simulink model "exp4_1"  (R2024b)
settings: Solver=VariableStepAuto  StartTime=0.0  StopTime=10  RelTol=1e-3
InitFcn:
  | Voc=32.9;
  | Iscn=8.21;
  | k=1.38e-23;
  | Ns=54;
  | Np=1;
  | G=524;
  | Gn=1000;
  | Kv=-0.1230;
  | Ki=0.0032;
  | T=301;
  | Tn=300;
  | q=1.6e-19;
  | I0n=9.85e-8;
  | Eg=1.12;
  | Ign=8.214;
  | Rs=0.221;
  | Rp=414.5;
  | a=1.0;
libraries: spsSeriesRLCBranchLib x6, spsVoltageMeasurementLib x4, spsCurrentMeasurementLib x3, spsDiodeLib x2, spsFirstOrderFilterLib x2, spsMeanLib x2, slpidlib x1, spsMosfetLib x1, spsControlledCurrentSourceLib x1, simulink x1, spspowerguiLib x1, spsPWMGeneratorDCDCLib x1
settings Model: Creator=palla  LastModifiedBy=palla

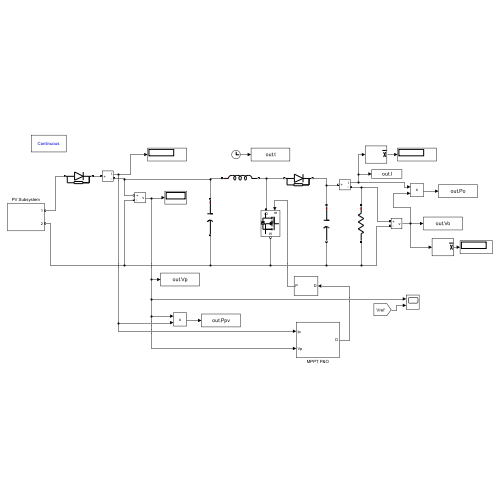
[thumbnail: Simulink's stored preview of the top-level diagram]
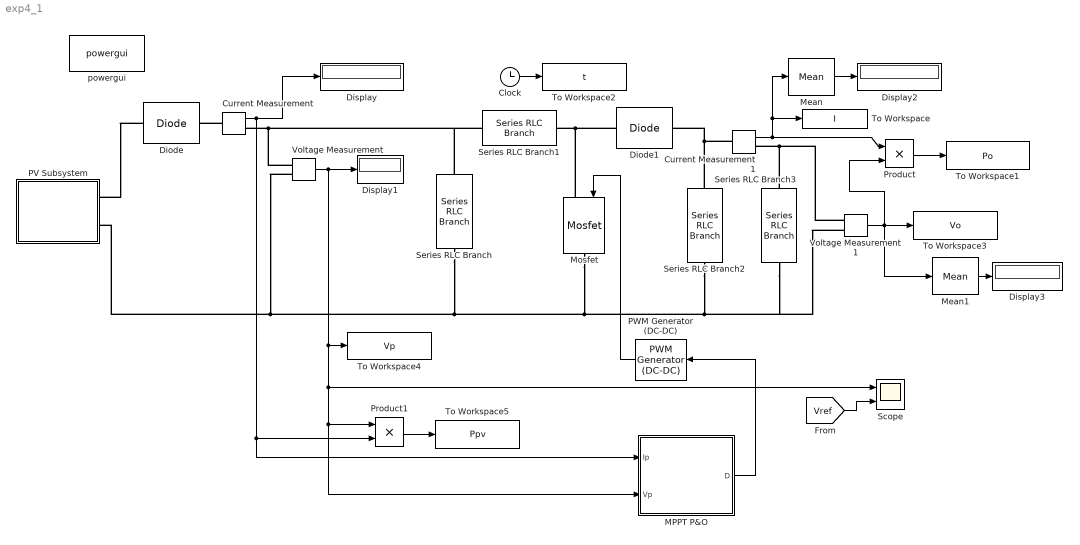
== system exp4_1 ==
  Clock : Clock
  Current Measurement : spsCurrentMeasurementLib/Current Measurement  PhasorSimulation=off  OutputType=Complex  PSBequivalent=0
  Current Measurement1 : spsCurrentMeasurementLib/Current Measurement  PhasorSimulation=off  OutputType=Complex  PSBequivalent=0
  Diode : spsDiodeLib/Diode  Ron=0.001  Lon=0  Vf=0.8  IC=0  UseSnubber=0  Rs=500  Cs=250e-9  Measurements=off
  Diode1 : spsDiodeLib/Diode  Ron=0.001  Lon=0  Vf=0.8  IC=0  UseSnubber=0  Rs=500  Cs=250e-9  Measurements=off
  Display{,1..3} (4 alike) : Display
  MPPT P&O : Subsystem
  Mean : spsMeanLib/Mean  Freq=60  Vinit=0  Ts=0
  Mean1 : spsMeanLib/Mean  Freq=60  Vinit=0  Ts=0
  Mosfet : spsMosfetLib/Mosfet  Ron=0.1  Lon=0  Rd=0.01  Vfd=0  IC=0  Rs=1e5  Cs=inf  Measurements=off
  PV Subsystem : Subsystem
  PWM Generator (DC-DC) : spsPWMGeneratorDCDCLib/PWM Generator (DC-DC)  Fsw=5000  Ts=0
  Product : Product
  Product1 : Product
  Scope : Scope  NumInputPorts=2
  Series RLC Branch : spsSeriesRLCBranchLib/Series RLC Branch  LConnTagsString=__new0  RConnTagsString=__new0  BranchType=C  Resistance=1  Inductance=1e-3  SetiL0=off  InitialCurrent=0  Capacitance=110e-6  Setx0=off  InitialVoltage=0  Measurements=None
  Series RLC Branch1 : spsSeriesRLCBranchLib/Series RLC Branch  LConnTagsString=__new0  RConnTagsString=__new0  BranchType=L  Resistance=1  Inductance=0.01025  SetiL0=off  InitialCurrent=0  Capacitance=1e-6  Setx0=off  InitialVoltage=0  Measurements=None
  Series RLC Branch2 : spsSeriesRLCBranchLib/Series RLC Branch  LConnTagsString=__new0  RConnTagsString=__new0  BranchType=C  Resistance=1  Inductance=1e-3  SetiL0=off  InitialCurrent=0  Capacitance=110e-6  Setx0=off  InitialVoltage=0  Measurements=None
  Series RLC Branch3 : spsSeriesRLCBranchLib/Series RLC Branch  LConnTagsString=__new0  RConnTagsString=__new0  BranchType=R  Resistance=25.5  Inductance=1e-3  SetiL0=off  InitialCurrent=0  Capacitance=1e-6  Setx0=off  InitialVoltage=0  Measurements=None
  To Workspace : ToWorkspace  VariableName=I  SampleTime=-1
  To Workspace1 : ToWorkspace  VariableName=Po  SampleTime=-1
  To Workspace2 : ToWorkspace  VariableName=t  SampleTime=-1
  To Workspace3 : ToWorkspace  VariableName=Vo  SampleTime=-1
  To Workspace4 : ToWorkspace  VariableName=Vp  SampleTime=-1
  To Workspace5 : ToWorkspace  VariableName=Ppv  SampleTime=-1
  Voltage Measurement : spsVoltageMeasurementLib/Voltage Measurement  PhasorSimulation=off  OutputType=Complex  PSBequivalent=0
  Voltage Measurement1 : spsVoltageMeasurementLib/Voltage Measurement  PhasorSimulation=off  OutputType=Complex  PSBequivalent=0
  powergui : sps_lib/powergui  Priority=1  SimulationMode=Continuous  SampleTime=50e-6  frequency=60  Iterations=50  frequencyindice=0  Pbase=100e6  ErrMax=1e-4  UnitsV=kV  UnitsW=MW  buscounter=0  FunctionMessages=off  echomessages=off  EnableUseOfTLC=off  CurrentSourceSwitches=off  DisableSnubberDevices=off  DisableRonSwitches=off  DisableVfSwitches=off  DisplayEquations=off  AutomaticDiscreteSolvers=off  SolverType=Tustin/Backward Euler (TBE)  Interpol=off  ExternalGateDelay=off  methode=off  Ts=100  x0status=blocks  SPID=on  SwTol=0  HookPort=off  NonlinearTolerance=1e-4  nMaxIteration=100  ContinueOnMaxIteration=off  RestoreLinks=warning  ResistiveCurrentMeasurement=off  Frange=[0:2:500]  Ylog=off  Xlog=on  ShowGrid=off  save=off  variable=ZData  structure=0  ZoomFFT=off  StartTime=0.0  cycles=1  DisplayStyle=1  fundamental=60  FreqAxis=off  MaxFrequency=1000  frequencyindicesteady=1  RmsSteady=1  display=off
  wires:
  Current Measurement/1 -> MPPT P&O/1(Ip), Product1/2, Display/1
  Voltage Measurement/1 -> MPPT P&O/2(Vp), Product1/1, Scope/1, To Workspace4/1, Display1/1
  PWM Generator (DC-DC)/1 -> Mosfet/1
  Current Measurement1/1 -> Mean/1, To Workspace/1, Product/1
  Mean/1 -> Display2/1
  Product/1 -> To Workspace1/1
  Clock/1 -> To Workspace2/1
  Voltage Measurement1/1 -> Product/2, Mean1/1, To Workspace3/1
  Mean1/1 -> Display3/1
  [Vref] -> Scope/2
  Product1/1 -> To Workspace5/1
  MPPT P&O/1(D) -> PWM Generator (DC-DC)/1
  connections:
  Diode/LConn1 -- PV Subsystem/LConn1
  Current Measurement/LConn1 -- Diode/RConn1
  Voltage Measurement/LConn1 -- Series RLC Branch1/LConn1 -- Series RLC Branch/LConn1 -- Current Measurement/RConn1
  Diode1/LConn1 -- Mosfet/LConn1 -- Series RLC Branch1/RConn1
  Mosfet/RConn1 -- Series RLC Branch3/RConn1 -- Voltage Measurement1/LConn2 -- Series RLC Branch2/RConn1 -- Series RLC Branch/RConn1 -- Voltage Measurement/LConn2 -- PV Subsystem/LConn2
  Series RLC Branch2/LConn1 -- Diode1/RConn1 -- Current Measurement1/LConn1
  Series RLC Branch3/LConn1 -- Voltage Measurement1/LConn1 -- Current Measurement1/RConn1

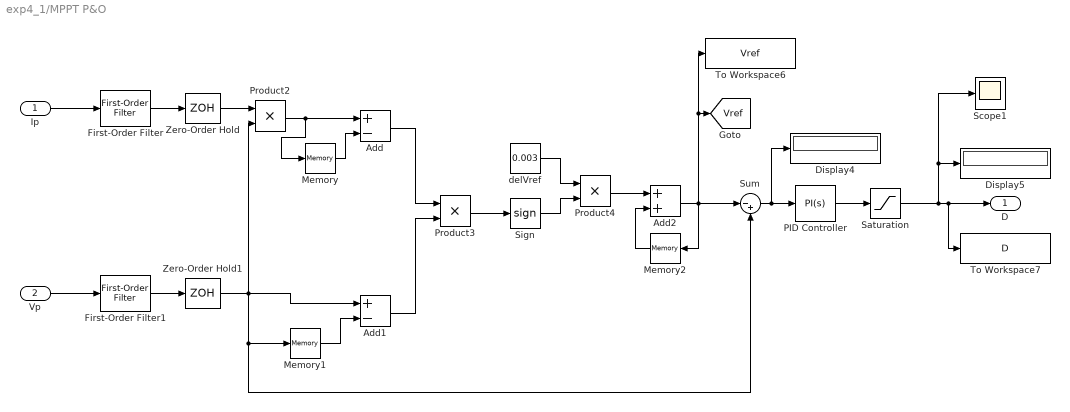
== system exp4_1/MPPT P&O ==
  Ip : Inport
  Vp : Inport  Port=2
  Add : Sum  Inputs=+-
  Add1 : Sum  Inputs=+-
  Add2 : Sum
  Display4 : Display
  Display5 : Display
  First-Order Filter : spsFirstOrderFilterLib/First-Order Filter  FilterType=Lowpass  Tc=10e-3  Ts=0  Initialize=on  Vac_Init=[0, 0, 60]  Vdc_Init=0  PlotResponse=off  FreqRange="[0,  200,  1]"
  First-Order Filter1 : spsFirstOrderFilterLib/First-Order Filter  FilterType=Lowpass  Tc=10e-3  Ts=0  Initialize=on  Vac_Init=[0, 0, 60]  Vdc_Init=0  PlotResponse=off  FreqRange="[0,  200,  1]"
  Memory : Memory
  Memory1 : Memory
  Memory2 : Memory
  PID Controller : slpidlib/PID Controller  Controller=PI  Form=Parallel  TimeDomain=Continuous-time  UseExternalTs=off  SampleTime=-1  IntegratorMethod=Forward Euler  FilterMethod=Forward Euler  ControllerParametersSource=internal  P=0.001  I=0.1  UseKiTs=off  D=0  UseExternalDerivativeSource=off  N=100  UseFilter=on  TunerSelectOption=Transfer Function Based (PID Tuner App)  InitialConditionSource=internal  InitialConditionForIntegrator=0  InitialConditionForFilter=0  DifferentiatorICPrevScaledInput=0  ExternalReset=none  TrackingMode=off  Kt=1  LimitOutput=off  SatLimitsSource=internal  UpperSaturationLimit=inf  LowerSaturationLimit=-inf  LinearizeAsGain=on  AntiWindupMode=none  Kb=1  LimitIntegrator=off  UpperIntegratorSaturationLimit=inf  LowerIntegratorSaturationLimit=-inf  POutMin=[]  POutMax=[]  IOutMin=[]  IOutMax=[]  DOutMin=[]  DOutMax=[]  NOutMin=[]  NOutMax=[]  SumOutMin=[]  SumOutMax=[]  SaturationOutMin=[]  SaturationOutMax=[]  PParamMin=[]  PParamMax=[]  IParamMin=[]  IParamMax=[]  DParamMin=[]  DParamMax=[]  NParamMin=[]  NParamMax=[]  KbParamMin=[]  KbParamMax=[]  KtParamMin=[]  KtParamMax=[]  KbOutMin=[]  KbOutMax=[]  KtOutMin=[]  KtOutMax=[]  IntegratorOutMin=[]  IntegratorOutMax=[]  FilterOutMin=[]  FilterOutMax=[]  SumI1OutMin=[]  SumI1OutMax=[]  SumI2OutMin=[]  SumI2OutMax=[]  SumI3OutMin=[]  SumI3OutMax=[]  SumI4OutMin=[]  SumI4OutMax=[]  SumDOutMin=[]  SumDOutMax=[]  DifferentiatorOutMin=[]  DifferentiatorOutMax=[]  FilterDiffOutCoefMin=[]  FilterDiffOutCoefMax=[]  ReciprocalOutMin=[]  ReciprocalOutMax=[]  SumDenOutMin=[]  SumDenOutMax=[]  SumNumOutMin=[]  SumNumOutMax=[]  DivideOutMin=[]  DivideOutMax=[]  UdiffTsProdOutMin=[]  UdiffTsProdOutMax=[]  NTsProdOutMin=[]  NTsProdOutMax=[]  UintegralTsProdOutMin=[]  UintegralTsProdOutMax=[]  UngainTsProdOutMin=[]  UngainTsProdOutMax=[]  ClampingZeroOutDataTypeStr=Inherit: Inherit via back propagation  ClampingZeroOutMin=[]  ClampingZeroOutMax=[]  FilterDenConstantOutDataTypeStr=Inherit: Inherit via back propagation  FilterDenConstantOutMin=[]  FilterDenConstantOutMax=[]  PCopyOutDataTypeStr=Inherit: Inherit via back propagation  PCopyOutMin=[]  PCopyOutMax=[]  NCopyOutDataTypeStr=Inherit: Inherit via back propagation  NCopyOutMin=[]  NCopyOutMax=[]  IntegratorContinuousStateAttributes=''  IntegratorStateMustResolveToSignalObject=off  IntegratorRTWStateStorageClass=Auto  FilterContinuousStateAttributes=''  FilterStateMustResolveToSignalObject=off  FilterRTWStateStorageClass=Auto  ParallelPVariant=InternalParameters  IdealPVariant=Disabled  IVariant=InternalParameters  DVariant=Disabled  IntegratorVariant=Continuous  SatVariant=Disabled  AWVariant=Passthrough  PCopyVariant=Disabled  TRVariant=Disabled  FdbkBlocksVariant=Forward  IdealPFdbkVariant=Disabled  SatFdbkVariant=Disabled  DerivativeFilterVariant=Disabled  NVariant=Disabled  NCopyVariant=Disabled_SignalSpec  FilterICVariant=Disabled  IntegratorICVariant=InternalICs  ExternalResetVariant=Disabled  TRSumVariant=Passthrough  SumFdbkVariant=Disabled  SumVariant=Sum_PI  TsampFilterVariant=InternalTs  TsampNgainVariant=Passthrough  TsampIntegralVariant=Disabled_SignalSpec  ExternalSaturationOutDataTypeStr=Inherit: Same as second input  DerivativeSourceVariant=Disabled  PreIntVariant=InternalPreInt
  Product2 : Product
  Product3 : Product
  Product4 : Product
  Saturation : Saturate  UpperLimit=1  LowerLimit=0
  Scope1 : Scope
  Sign : Signum
  Sum : Sum  Inputs=|-+
  To Workspace6 : ToWorkspace  VariableName=Vref  SaveFormat=Timeseries  SampleTime=-1
  To Workspace7 : ToWorkspace  VariableName=D  SaveFormat=Timeseries  SampleTime=-1
  Zero-Order Hold : ZeroOrderHold  SampleTime=-1
  Zero-Order Hold1 : ZeroOrderHold  SampleTime=-1
  delVref : Constant  Value=0.003
  D : Outport
  tag scope: Vref=global
  wires:
  Sign/1 -> Product4/2
  Vp/1 -> First-Order Filter1/1
  Product3/1 -> Sign/1
  Add2/1 -> Memory2/1, To Workspace6/1, [Vref], Sum/1
  First-Order Filter/1 -> Zero-Order Hold/1
  Saturation/1 -> Scope1/1, Display5/1, D/1, To Workspace7/1
  Zero-Order Hold1/1 -> Add1/1, Sum/2, Memory1/1, Product2/2
  Product2/1 -> Memory/1, Add/1
  Memory1/1 -> Add1/2
  First-Order Filter1/1 -> Zero-Order Hold1/1
  delVref/1 -> Product4/1
  Ip/1 -> First-Order Filter/1
  Memory/1 -> Add/2
  Add1/1 -> Product3/2
  Product4/1 -> Add2/1
  Add/1 -> Product3/1
  Zero-Order Hold/1 -> Product2/1
  Memory2/1 -> Add2/2
  PID Controller/1 -> Saturation/1
  Sum/1 -> Display4/1, PID Controller/1

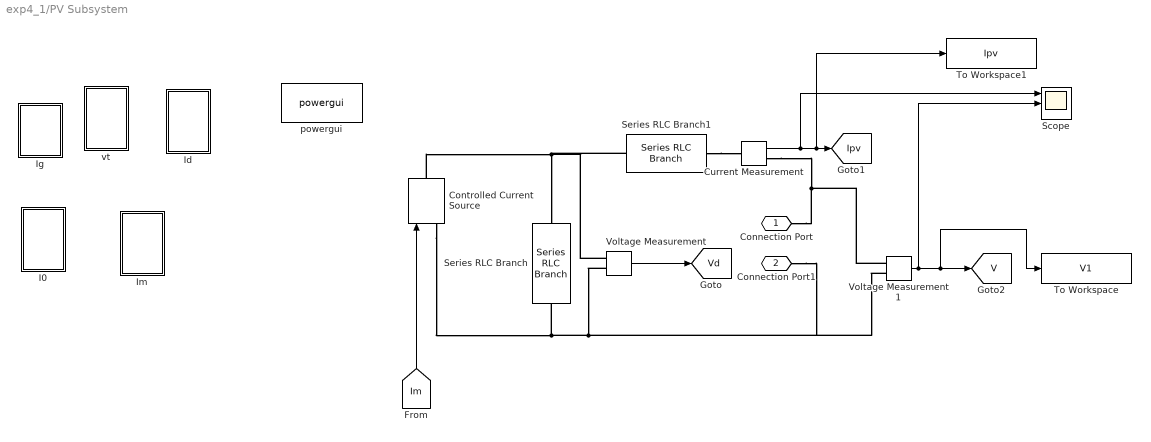
== system exp4_1/PV Subsystem ==
  Controlled Current Source : spsControlledCurrentSourceLib/Controlled Current Source  Initialize=on  Source_Type=AC  Amplitude=0  Phase=0  Frequency=0  Measurements=None
  Current Measurement : spsCurrentMeasurementLib/Current Measurement  PhasorSimulation=off  OutputType=Complex  PSBequivalent=0
  I0 : Subsystem
  Id : Subsystem
  Ig : Subsystem
  Im : Subsystem
  Scope : Scope  NumInputPorts=3
  Series RLC Branch : spsSeriesRLCBranchLib/Series RLC Branch  LConnTagsString=__new0  RConnTagsString=__new0  BranchType=R  Resistance=Rp  Inductance=1e-3  SetiL0=off  InitialCurrent=0  Capacitance=1e-6  Setx0=off  InitialVoltage=0  Measurements=None
  Series RLC Branch1 : spsSeriesRLCBranchLib/Series RLC Branch  LConnTagsString=__new0  RConnTagsString=__new0  BranchType=R  Resistance=Rs  Inductance=1e-3  SetiL0=off  InitialCurrent=0  Capacitance=1e-6  Setx0=off  InitialVoltage=0  Measurements=None
  To Workspace : ToWorkspace  VariableName=V1  SampleTime=-1
  To Workspace1 : ToWorkspace  VariableName=Ipv  SampleTime=-1
  Voltage Measurement : spsVoltageMeasurementLib/Voltage Measurement  PhasorSimulation=off  OutputType=Complex  PSBequivalent=0
  Voltage Measurement1 : spsVoltageMeasurementLib/Voltage Measurement  PhasorSimulation=off  OutputType=Complex  PSBequivalent=0
  powergui : spspowerguiLib/powergui  Priority=1  SimulationMode=Continuous  SampleTime=50e-6  frequency=60  Iterations=50  frequencyindice=0  Pbase=100e6  ErrMax=1e-4  UnitsV=kV  UnitsW=MW  buscounter=0  FunctionMessages=off  echomessages=off  EnableUseOfTLC=off  CurrentSourceSwitches=off  DisableSnubberDevices=off  DisableRonSwitches=off  DisableVfSwitches=off  DisplayEquations=off  AutomaticDiscreteSolvers=off  SolverType=Tustin/Backward Euler (TBE)  Interpol=off  ExternalGateDelay=off  methode=off  Ts=100  x0status=blocks  SPID=on  SwTol=0  HookPort=off  NonlinearTolerance=1e-4  nMaxIteration=100  ContinueOnMaxIteration=off  RestoreLinks=warning  ResistiveCurrentMeasurement=off  Frange=[0:2:500]  Ylog=off  Xlog=on  ShowGrid=off  save=off  variable=ZData  structure=0  ZoomFFT=off  StartTime=0.0  cycles=1  DisplayStyle=1  fundamental=60  FreqAxis=off  MaxFrequency=1000  frequencyindicesteady=1  RmsSteady=1  display=off
  vt : Subsystem
  Connection Port : PMIOPort  Side=Left
  Connection Port1 : PMIOPort  Port=2  Side=Left
  tag scope: Ipv=global, V=global, Vd=global
  wires:
  Voltage Measurement/1 -> [Vd]
  Current Measurement/1 -> Scope/1, To Workspace1/1, [Ipv]
  [Im] -> Controlled Current Source/1
  Voltage Measurement1/1 -> Scope/2, To Workspace/1, [V]
  connections:
  Controlled Current Source/LConn1 -- Connection Port1/RConn1 -- Voltage Measurement1/LConn2 -- Voltage Measurement/LConn2 -- Series RLC Branch/RConn1
  Controlled Current Source/RConn1 -- Voltage Measurement/LConn1 -- Series RLC Branch1/RConn1 -- Series RLC Branch/LConn1
  Current Measurement/RConn1 -- Connection Port/RConn1 -- Voltage Measurement1/LConn1
  Series RLC Branch1/LConn1 -- Current Measurement/LConn1

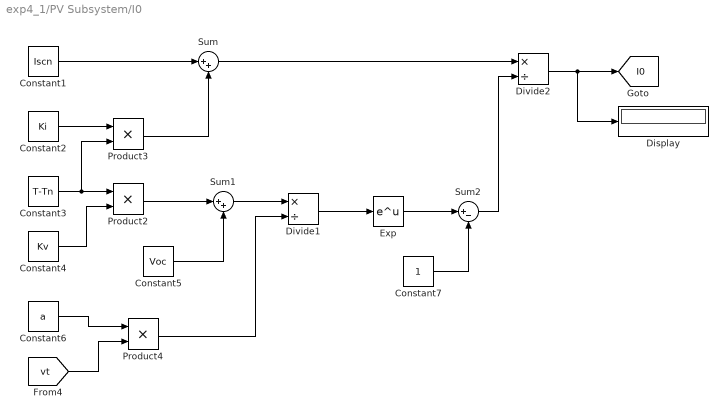
== system exp4_1/PV Subsystem/I0 ==
  Constant1 : Constant  Value=Iscn
  Constant2 : Constant  Value=Ki
  Constant3 : Constant  Value=T-Tn
  Constant4 : Constant  Value=Kv
  Constant5 : Constant  Value=Voc
  Constant6 : Constant  Value=a
  Constant7 : Constant
  Display : Display
  Divide1 : Product  Inputs=*/
  Divide2 : Product  Inputs=*/
  Exp : Math
  Product2 : Product
  Product3 : Product
  Product4 : Product
  Sum : Sum  Inputs=|++
  Sum1 : Sum  Inputs=|++
  Sum2 : Sum  Inputs=|+-
  tag scope: I0=global
  wires:
  Constant2/1 -> Product3/1
  Sum/1 -> Divide2/1
  Divide2/1 -> Display/1, [I0]
  Divide1/1 -> Exp/1
  Constant6/1 -> Product4/1
  Sum1/1 -> Divide1/1
  [vt] -> Product4/2
  Product4/1 -> Divide1/2
  Constant4/1 -> Product2/2
  Constant5/1 -> Sum1/2
  Sum2/1 -> Divide2/2
  Constant1/1 -> Sum/1
  Product2/1 -> Sum1/1
  Product3/1 -> Sum/2
  Constant3/1 -> Product3/2, Product2/1
  Exp/1 -> Sum2/1
  Constant7/1 -> Sum2/2

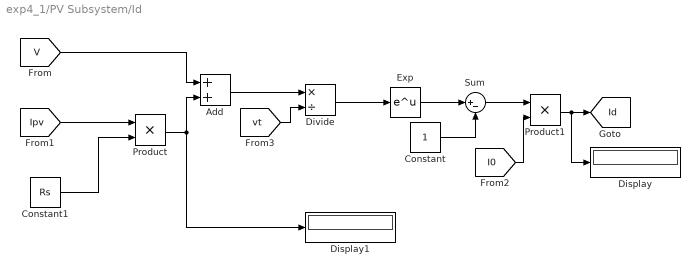
== system exp4_1/PV Subsystem/Id ==
  Add : Sum
  Constant : Constant
  Constant1 : Constant  Value=Rs
  Display : Display
  Display1 : Display
  Divide : Product  Inputs=*/
  Exp : Math
  Product : Product
  Product1 : Product
  Sum : Sum  Inputs=|+-
  tag scope: Id=global
  wires:
  Product1/1 -> Display/1, [Id]
  Constant1/1 -> Product/2
  Product/1 -> Add/2, Display1/1
  [I0] -> Product1/2
  [Ipv] -> Product/1
  Exp/1 -> Sum/1
  Constant/1 -> Sum/2
  Sum/1 -> Product1/1
  [V] -> Add/1
  Add/1 -> Divide/1
  [vt] -> Divide/2
  Divide/1 -> Exp/1

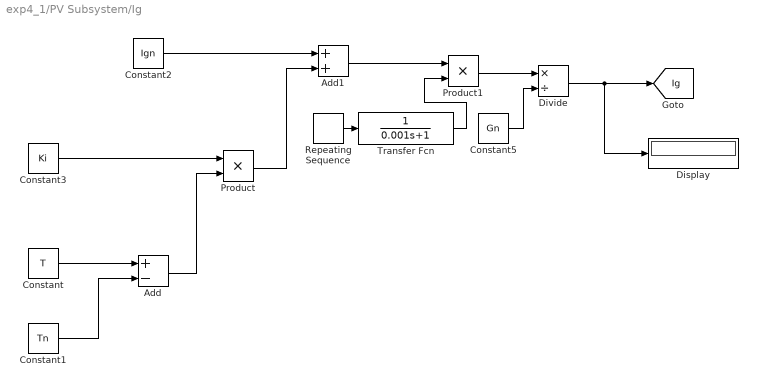
== system exp4_1/PV Subsystem/Ig ==
  Add : Sum  Inputs=+-
  Add1 : Sum
  Constant : Constant  Value=T
  Constant1 : Constant  Value=Tn
  Constant2 : Constant  Value=Ign
  Constant3 : Constant  Value=Ki
  Constant5 : Constant  Value=Gn
  Display : Display
  Divide : Product  Inputs=*/
  Product : Product
  Product1 : Product
  Repeating Sequence : simulink/Sources/Repeating Sequence  rep_seq_t=[0 3 3.1 7 7.1 10]  rep_seq_y=[640 640 810 810 980 980]
  Transfer Fcn : TransferFcn  Denominator=[0.001 1]
  tag scope: Ig=global
  wires:
  Constant2/1 -> Add1/1
  Constant1/1 -> Add/2
  Add/1 -> Product/2
  Constant3/1 -> Product/1
  Add1/1 -> Product1/1
  Constant5/1 -> Divide/2
  Product/1 -> Add1/2
  Constant/1 -> Add/1
  Product1/1 -> Divide/1
  Divide/1 -> Display/1, [Ig]
  Transfer Fcn/1 -> Product1/2
  Repeating Sequence/1 -> Transfer Fcn/1

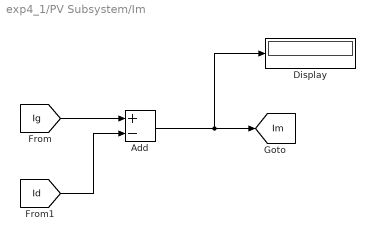
== system exp4_1/PV Subsystem/Im ==
  Add : Sum  Inputs=+-
  Display : Display
  tag scope: Im=global
  wires:
  Add/1 -> Display/1, [Im]
  [Id] -> Add/2
  [Ig] -> Add/1

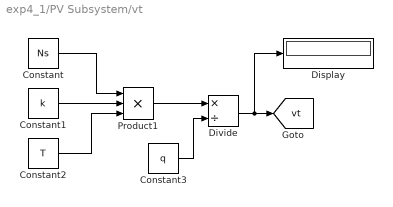
== system exp4_1/PV Subsystem/vt ==
  Constant : Constant  Value=Ns
  Constant1 : Constant  Value=k
  Constant2 : Constant  Value=T
  Constant3 : Constant  Value=q
  Display : Display
  Divide : Product  Inputs=*/
  Product1 : Product  Inputs=3
  tag scope: vt=global
  wires:
  Product1/1 -> Divide/1
  Constant3/1 -> Divide/2
  Constant2/1 -> Product1/3
  Constant/1 -> Product1/1
  Divide/1 -> Display/1, [vt]
  Constant1/1 -> Product1/2
